simulink model "TST_Rail_BlkShtCtl"  (R2016b)
settings: Solver=FixedStepDiscrete  StartTime=0.0  StopTime=simTime  FixedStep=sampleTime  RelTol=1e-3
values from neighbouring files (symbols this model uses):
  testCase = 1    [initTST_Rail_BlkShtCtl_001.m]    (also in initTST_Rail_BlkShtCtl_002.m = 2; initTST_Rail_BlkShtCtl_003.m = 3)
libraries: simulink x7, UnitTest_Lib x3
settings Model: Creator=zhengjinyan  LastModifiedBy=zhengjinyan
settings DebuggingCC: SignalRangeChecking=error

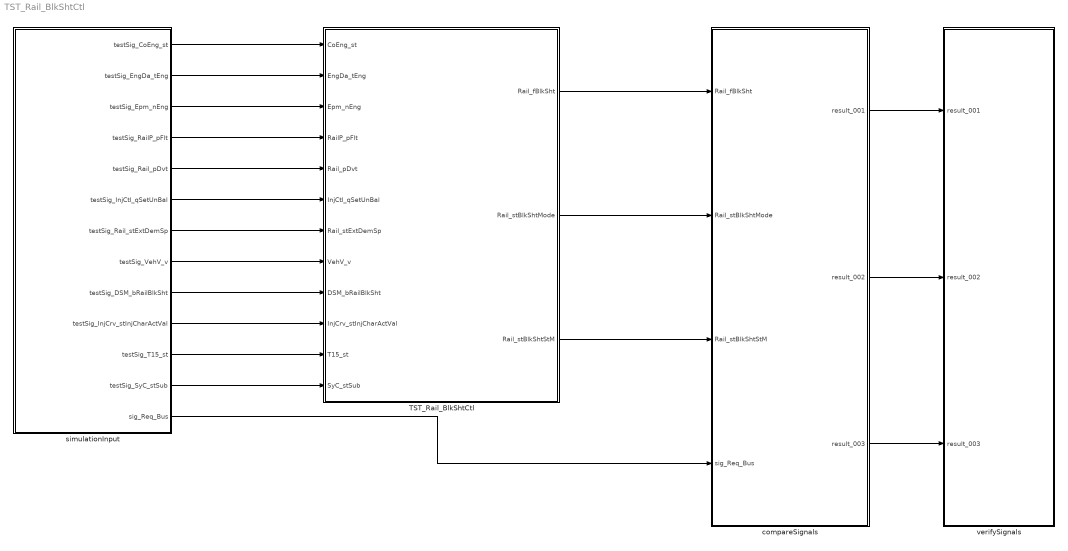
== system TST_Rail_BlkShtCtl ==
  TST_Rail_BlkShtCtl : Subsystem
  compareSignals : Subsystem
  simulationInput : Subsystem
  verifySignals : Subsystem
  wires:
  simulationInput/1(testSig_CoEng_st) -> TST_Rail_BlkShtCtl/1(CoEng_st)
  simulationInput/2(testSig_EngDa_tEng) -> TST_Rail_BlkShtCtl/2(EngDa_tEng)
  simulationInput/3(testSig_Epm_nEng) -> TST_Rail_BlkShtCtl/3(Epm_nEng)
  simulationInput/4(testSig_RailP_pFlt) -> TST_Rail_BlkShtCtl/4(RailP_pFlt)
  simulationInput/5(testSig_Rail_pDvt) -> TST_Rail_BlkShtCtl/5(Rail_pDvt)
  simulationInput/6(testSig_InjCtl_qSetUnBal) -> TST_Rail_BlkShtCtl/6(InjCtl_qSetUnBal)
  simulationInput/7(testSig_Rail_stExtDemSp) -> TST_Rail_BlkShtCtl/7(Rail_stExtDemSp)
  simulationInput/8(testSig_VehV_v) -> TST_Rail_BlkShtCtl/8(VehV_v)
  simulationInput/9(testSig_DSM_bRailBlkSht) -> TST_Rail_BlkShtCtl/9(DSM_bRailBlkSht)
  simulationInput/10(testSig_InjCrv_stInjCharActVal) -> TST_Rail_BlkShtCtl/10(InjCrv_stInjCharActVal)
  simulationInput/11(testSig_T15_st) -> TST_Rail_BlkShtCtl/11(T15_st)
  simulationInput/12(testSig_SyC_stSub) -> TST_Rail_BlkShtCtl/12(SyC_stSub)
  TST_Rail_BlkShtCtl/1(Rail_fBlkSht) -> compareSignals/1(Rail_fBlkSht)
  TST_Rail_BlkShtCtl/2(Rail_stBlkShtMode) -> compareSignals/2(Rail_stBlkShtMode)
  TST_Rail_BlkShtCtl/3(Rail_stBlkShtStM) -> compareSignals/3(Rail_stBlkShtStM)
  simulationInput/13(sig_Req_Bus) -> compareSignals/4(sig_Req_Bus)
  compareSignals/1(result_001) -> verifySignals/1(result_001)
  compareSignals/2(result_002) -> verifySignals/2(result_002)
  compareSignals/3(result_003) -> verifySignals/3(result_003)

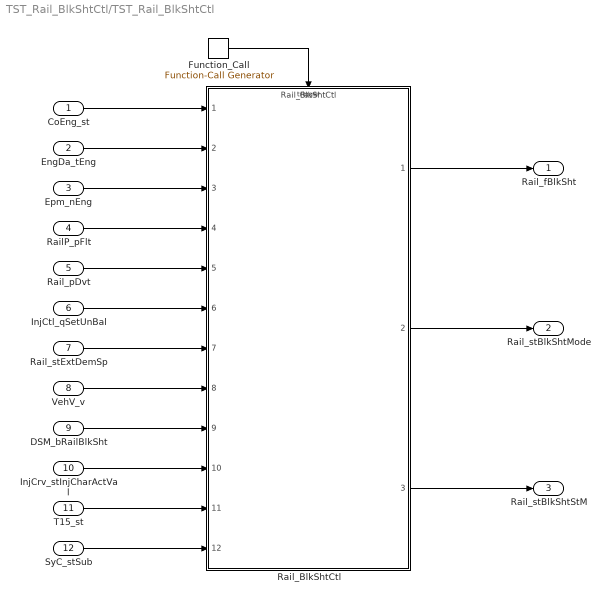
== system TST_Rail_BlkShtCtl/TST_Rail_BlkShtCtl ==
  CoEng_st : Inport
  EngDa_tEng : Inport  Port=2
  Epm_nEng : Inport  Port=3
  RailP_pFlt : Inport  Port=4
  Rail_pDvt : Inport  Port=5
  InjCtl_qSetUnBal : Inport  Port=6
  Rail_stExtDemSp : Inport  Port=7
  VehV_v : Inport  Port=8
  DSM_bRailBlkSht : Inport  Port=9
  InjCrv_stInjCharActVal : Inport  Port=10
  T15_st : Inport  Port=11
  SyC_stSub : Inport  Port=12
  Function_Call : simulink/Ports & Subsystems/Function-Call Generator  sample_time=sampleTime  numberOfIterations=1
  Rail_BlkShtCtl : ModelReference  ModelNameDialog=Rail_BlkShtCtl  SimulationMode=Normal  ModelReferenceVersion=1.164  TriggerPortName=function  TriggerPortTriggerType=function-call  TriggerPortStatesWhenEnabling=held
  Rail_fBlkSht : Outport
  Rail_stBlkShtMode : Outport  Port=2
  Rail_stBlkShtStM : Outport  Port=3
  wires:
  Function_Call/1 -> Rail_BlkShtCtl/Trigger
  CoEng_st/1 -> Rail_BlkShtCtl/1
  EngDa_tEng/1 -> Rail_BlkShtCtl/2
  Epm_nEng/1 -> Rail_BlkShtCtl/3
  RailP_pFlt/1 -> Rail_BlkShtCtl/4
  Rail_pDvt/1 -> Rail_BlkShtCtl/5
  InjCtl_qSetUnBal/1 -> Rail_BlkShtCtl/6
  Rail_stExtDemSp/1 -> Rail_BlkShtCtl/7
  VehV_v/1 -> Rail_BlkShtCtl/8
  DSM_bRailBlkSht/1 -> Rail_BlkShtCtl/9
  InjCrv_stInjCharActVal/1 -> Rail_BlkShtCtl/10
  T15_st/1 -> Rail_BlkShtCtl/11
  SyC_stSub/1 -> Rail_BlkShtCtl/12
  Rail_BlkShtCtl/1 -> Rail_fBlkSht/1
  Rail_BlkShtCtl/2 -> Rail_stBlkShtMode/1
  Rail_BlkShtCtl/3 -> Rail_stBlkShtStM/1

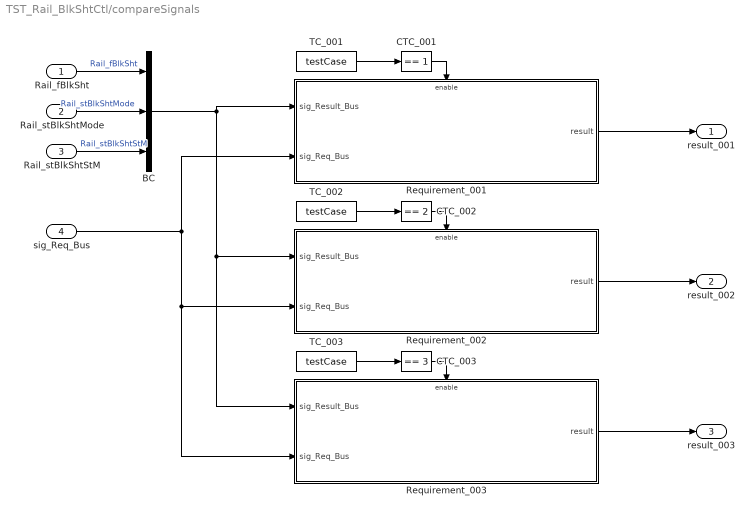
== system TST_Rail_BlkShtCtl/compareSignals ==
  Rail_fBlkSht : Inport
  Rail_stBlkShtMode : Inport  Port=2
  Rail_stBlkShtStM : Inport  Port=3
  sig_Req_Bus : Inport  Port=4
  BC : BusCreator  Inputs=3
  CTC_001 : simulink/Logic and Bit Operations/Compare To Constant  relop===  const=1  OutDataTypeStr=boolean
  CTC_002 : simulink/Logic and Bit Operations/Compare To Constant  relop===  const=2  OutDataTypeStr=boolean
  CTC_003 : simulink/Logic and Bit Operations/Compare To Constant  relop===  const=3  OutDataTypeStr=boolean
  Requirement_001 : Subsystem
  Requirement_002 : Subsystem
  Requirement_003 : Subsystem
  TC_001 : Constant  Value=testCase
  TC_002 : Constant  Value=testCase
  TC_003 : Constant  Value=testCase
  result_001 : Outport
  result_002 : Outport  Port=2
  result_003 : Outport  Port=3
  wires:
  Rail_fBlkSht/1 -> BC/1  "Rail_fBlkSht"
  Rail_stBlkShtMode/1 -> BC/2  "Rail_stBlkShtMode"
  Rail_stBlkShtStM/1 -> BC/3  "Rail_stBlkShtStM"
  TC_001/1 -> CTC_001/1
  CTC_001/1 -> Requirement_001/Enable
  sig_Req_Bus/1 -> Requirement_002/2(sig_Req_Bus), Requirement_003/2(sig_Req_Bus), Requirement_001/2(sig_Req_Bus)
  BC/1 -> Requirement_002/1(sig_Result_Bus), Requirement_003/1(sig_Result_Bus), Requirement_001/1(sig_Result_Bus)
  Requirement_001/1(result) -> result_001/1
  TC_002/1 -> CTC_002/1
  CTC_002/1 -> Requirement_002/Enable
  Requirement_002/1(result) -> result_002/1
  TC_003/1 -> CTC_003/1
  CTC_003/1 -> Requirement_003/Enable
  Requirement_003/1(result) -> result_003/1

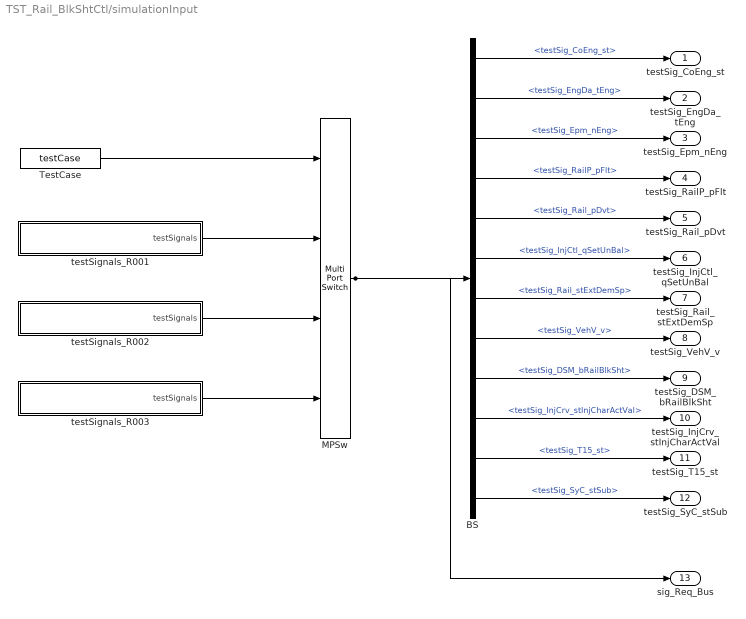
== system TST_Rail_BlkShtCtl/simulationInput ==
  BS : BusSelector  OutputSignals=testSig_CoEng_st,testSig_EngDa_tEng,testSig_Epm_nEng,testSig_RailP_pFlt,testSig_Rail_pDvt,testSig_InjCtl_qSetUnBal,testSig_Rail_stExtDemSp,testSig_VehV_v,testSig_DSM_bRailBlkSht,testSig_InjCrv_stInjCharActVal,testSig_T15_st,testSig_SyC_stSub
  MPSw : MultiPortSwitch  SaturateOnIntegerOverflow=on  InputSameDT=on
  TestCase : Constant  Value=testCase
  testSignals_R001 : Subsystem
  testSignals_R002 : Subsystem
  testSignals_R003 : Subsystem
  testSig_CoEng_st : Outport
  testSig_EngDa_tEng : Outport  Port=2
  testSig_Epm_nEng : Outport  Port=3
  testSig_RailP_pFlt : Outport  Port=4
  testSig_Rail_pDvt : Outport  Port=5
  testSig_InjCtl_qSetUnBal : Outport  Port=6
  testSig_Rail_stExtDemSp : Outport  Port=7
  testSig_VehV_v : Outport  Port=8
  testSig_DSM_bRailBlkSht : Outport  Port=9
  testSig_InjCrv_stInjCharActVal : Outport  Port=10
  testSig_T15_st : Outport  Port=11
  testSig_SyC_stSub : Outport  Port=12
  sig_Req_Bus : Outport  Port=13
  wires:
  BS/1 -> testSig_CoEng_st/1  "<testSig_CoEng_st>"
  BS/2 -> testSig_EngDa_tEng/1  "<testSig_EngDa_tEng>"
  BS/3 -> testSig_Epm_nEng/1  "<testSig_Epm_nEng>"
  BS/4 -> testSig_RailP_pFlt/1  "<testSig_RailP_pFlt>"
  BS/5 -> testSig_Rail_pDvt/1  "<testSig_Rail_pDvt>"
  BS/6 -> testSig_InjCtl_qSetUnBal/1  "<testSig_InjCtl_qSetUnBal>"
  BS/7 -> testSig_Rail_stExtDemSp/1  "<testSig_Rail_stExtDemSp>"
  BS/8 -> testSig_VehV_v/1  "<testSig_VehV_v>"
  BS/9 -> testSig_DSM_bRailBlkSht/1  "<testSig_DSM_bRailBlkSht>"
  BS/10 -> testSig_InjCrv_stInjCharActVal/1  "<testSig_InjCrv_stInjCharActVal>"
  BS/11 -> testSig_T15_st/1  "<testSig_T15_st>"
  BS/12 -> testSig_SyC_stSub/1  "<testSig_SyC_stSub>"
  MPSw/1 -> BS/1, sig_Req_Bus/1
  TestCase/1 -> MPSw/1
  testSignals_R001/1(testSignals) -> MPSw/2
  testSignals_R002/1(testSignals) -> MPSw/3
  testSignals_R003/1(testSignals) -> MPSw/4

== system TST_Rail_BlkShtCtl/verifySignals ==
  result_001 : Inport
  result_002 : Inport  Port=2
  result_003 : Inport  Port=3
  Assertion_001 : Assertion  Enabled=off
  Assertion_002 : Assertion  Enabled=off
  Assertion_003 : Assertion  Enabled=off
  wires:
  result_001/1 -> Assertion_001/1
  result_002/1 -> Assertion_002/1
  result_003/1 -> Assertion_003/1

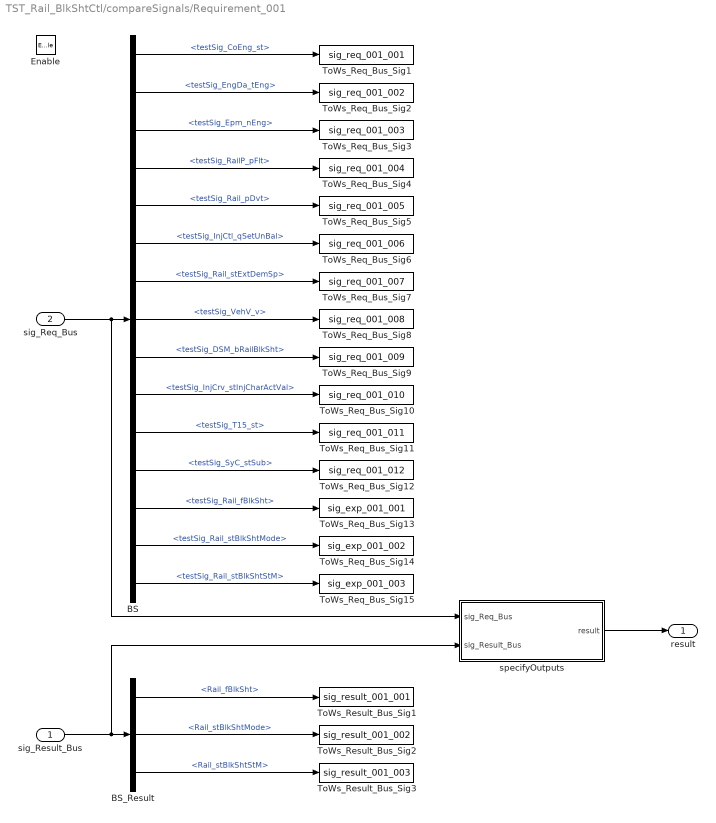
== system TST_Rail_BlkShtCtl/compareSignals/Requirement_001 ==
  sig_Result_Bus : Inport
  sig_Req_Bus : Inport  Port=2
  Enable : EnablePort
  BS : BusSelector  OutputSignals=testSig_CoEng_st,testSig_EngDa_tEng,testSig_Epm_nEng,testSig_RailP_pFlt,testSig_Rail_pDvt,testSig_InjCtl_qSetUnBal,testSig_Rail_stExtDemSp,testSig_VehV_v,testSig_DSM_bRailBlkSht,testSig_InjCrv_stInjCharActVal,testSig_T15_st,testSig_SyC_stSub,testSig_Rail_fBlkSht,testSig_Rail_stBlkShtMode,testSig_Rail_stBlkShtStM
  BS_Result : BusSelector  OutputSignals=Rail_fBlkSht,Rail_stBlkShtMode,Rail_stBlkShtStM
  ToWs_Req_Bus_Sig1 : ToWorkspace  VariableName=sig_req_001_001  SaveFormat=Structure With Time
  ToWs_Req_Bus_Sig10 : ToWorkspace  VariableName=sig_req_001_010  SaveFormat=Structure With Time
  ToWs_Req_Bus_Sig11 : ToWorkspace  VariableName=sig_req_001_011  SaveFormat=Structure With Time
  ToWs_Req_Bus_Sig12 : ToWorkspace  VariableName=sig_req_001_012  SaveFormat=Structure With Time
  ToWs_Req_Bus_Sig13 : ToWorkspace  VariableName=sig_exp_001_001  SaveFormat=Structure With Time
  ToWs_Req_Bus_Sig14 : ToWorkspace  VariableName=sig_exp_001_002  SaveFormat=Structure With Time
  ToWs_Req_Bus_Sig15 : ToWorkspace  VariableName=sig_exp_001_003  SaveFormat=Structure With Time
  ToWs_Req_Bus_Sig2 : ToWorkspace  VariableName=sig_req_001_002  SaveFormat=Structure With Time
  ToWs_Req_Bus_Sig3 : ToWorkspace  VariableName=sig_req_001_003  SaveFormat=Structure With Time
  ToWs_Req_Bus_Sig4 : ToWorkspace  VariableName=sig_req_001_004  SaveFormat=Structure With Time
  ToWs_Req_Bus_Sig5 : ToWorkspace  VariableName=sig_req_001_005  SaveFormat=Structure With Time
  ToWs_Req_Bus_Sig6 : ToWorkspace  VariableName=sig_req_001_006  SaveFormat=Structure With Time
  ToWs_Req_Bus_Sig7 : ToWorkspace  VariableName=sig_req_001_007  SaveFormat=Structure With Time
  ToWs_Req_Bus_Sig8 : ToWorkspace  VariableName=sig_req_001_008  SaveFormat=Structure With Time
  ToWs_Req_Bus_Sig9 : ToWorkspace  VariableName=sig_req_001_009  SaveFormat=Structure With Time
  ToWs_Result_Bus_Sig1 : ToWorkspace  VariableName=sig_result_001_001  SaveFormat=Structure With Time
  ToWs_Result_Bus_Sig2 : ToWorkspace  VariableName=sig_result_001_002  SaveFormat=Structure With Time
  ToWs_Result_Bus_Sig3 : ToWorkspace  VariableName=sig_result_001_003  SaveFormat=Structure With Time
  specifyOutputs : Subsystem
  result : Outport
  wires:
  sig_Req_Bus/1 -> BS/1, specifyOutputs/1(sig_Req_Bus)
  BS/1 -> ToWs_Req_Bus_Sig1/1  "<testSig_CoEng_st>"
  BS/2 -> ToWs_Req_Bus_Sig2/1  "<testSig_EngDa_tEng>"
  BS/3 -> ToWs_Req_Bus_Sig3/1  "<testSig_Epm_nEng>"
  BS/4 -> ToWs_Req_Bus_Sig4/1  "<testSig_RailP_pFlt>"
  BS/5 -> ToWs_Req_Bus_Sig5/1  "<testSig_Rail_pDvt>"
  BS/6 -> ToWs_Req_Bus_Sig6/1  "<testSig_InjCtl_qSetUnBal>"
  BS/7 -> ToWs_Req_Bus_Sig7/1  "<testSig_Rail_stExtDemSp>"
  BS/8 -> ToWs_Req_Bus_Sig8/1  "<testSig_VehV_v>"
  BS/9 -> ToWs_Req_Bus_Sig9/1  "<testSig_DSM_bRailBlkSht>"
  BS/10 -> ToWs_Req_Bus_Sig10/1  "<testSig_InjCrv_stInjCharActVal>"
  BS/11 -> ToWs_Req_Bus_Sig11/1  "<testSig_T15_st>"
  BS/12 -> ToWs_Req_Bus_Sig12/1  "<testSig_SyC_stSub>"
  BS/13 -> ToWs_Req_Bus_Sig13/1  "<testSig_Rail_fBlkSht>"
  BS/14 -> ToWs_Req_Bus_Sig14/1  "<testSig_Rail_stBlkShtMode>"
  BS/15 -> ToWs_Req_Bus_Sig15/1  "<testSig_Rail_stBlkShtStM>"
  sig_Result_Bus/1 -> BS_Result/1, specifyOutputs/2(sig_Result_Bus)
  BS_Result/1 -> ToWs_Result_Bus_Sig1/1  "<Rail_fBlkSht>"
  BS_Result/2 -> ToWs_Result_Bus_Sig2/1  "<Rail_stBlkShtMode>"
  BS_Result/3 -> ToWs_Result_Bus_Sig3/1  "<Rail_stBlkShtStM>"
  specifyOutputs/1(result) -> result/1

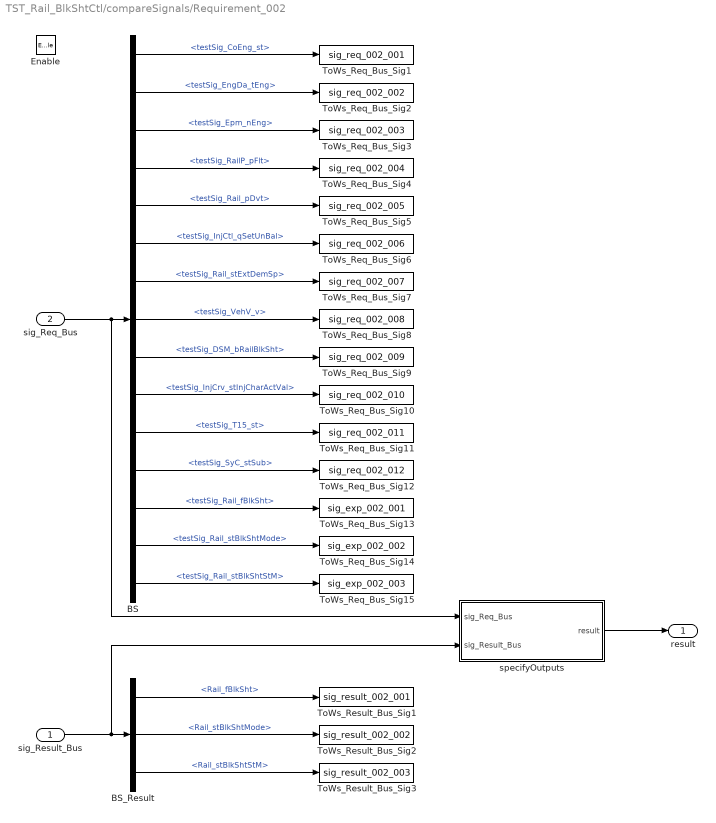
== system TST_Rail_BlkShtCtl/compareSignals/Requirement_002 ==
  sig_Result_Bus : Inport
  sig_Req_Bus : Inport  Port=2
  Enable : EnablePort
  BS : BusSelector  OutputSignals=testSig_CoEng_st,testSig_EngDa_tEng,testSig_Epm_nEng,testSig_RailP_pFlt,testSig_Rail_pDvt,testSig_InjCtl_qSetUnBal,testSig_Rail_stExtDemSp,testSig_VehV_v,testSig_DSM_bRailBlkSht,testSig_InjCrv_stInjCharActVal,testSig_T15_st,testSig_SyC_stSub,testSig_Rail_fBlkSht,testSig_Rail_stBlkShtMode,testSig_Rail_stBlkShtStM
  BS_Result : BusSelector  OutputSignals=Rail_fBlkSht,Rail_stBlkShtMode,Rail_stBlkShtStM
  ToWs_Req_Bus_Sig1 : ToWorkspace  VariableName=sig_req_002_001  SaveFormat=Structure With Time
  ToWs_Req_Bus_Sig10 : ToWorkspace  VariableName=sig_req_002_010  SaveFormat=Structure With Time
  ToWs_Req_Bus_Sig11 : ToWorkspace  VariableName=sig_req_002_011  SaveFormat=Structure With Time
  ToWs_Req_Bus_Sig12 : ToWorkspace  VariableName=sig_req_002_012  SaveFormat=Structure With Time
  ToWs_Req_Bus_Sig13 : ToWorkspace  VariableName=sig_exp_002_001  SaveFormat=Structure With Time
  ToWs_Req_Bus_Sig14 : ToWorkspace  VariableName=sig_exp_002_002  SaveFormat=Structure With Time
  ToWs_Req_Bus_Sig15 : ToWorkspace  VariableName=sig_exp_002_003  SaveFormat=Structure With Time
  ToWs_Req_Bus_Sig2 : ToWorkspace  VariableName=sig_req_002_002  SaveFormat=Structure With Time
  ToWs_Req_Bus_Sig3 : ToWorkspace  VariableName=sig_req_002_003  SaveFormat=Structure With Time
  ToWs_Req_Bus_Sig4 : ToWorkspace  VariableName=sig_req_002_004  SaveFormat=Structure With Time
  ToWs_Req_Bus_Sig5 : ToWorkspace  VariableName=sig_req_002_005  SaveFormat=Structure With Time
  ToWs_Req_Bus_Sig6 : ToWorkspace  VariableName=sig_req_002_006  SaveFormat=Structure With Time
  ToWs_Req_Bus_Sig7 : ToWorkspace  VariableName=sig_req_002_007  SaveFormat=Structure With Time
  ToWs_Req_Bus_Sig8 : ToWorkspace  VariableName=sig_req_002_008  SaveFormat=Structure With Time
  ToWs_Req_Bus_Sig9 : ToWorkspace  VariableName=sig_req_002_009  SaveFormat=Structure With Time
  ToWs_Result_Bus_Sig1 : ToWorkspace  VariableName=sig_result_002_001  SaveFormat=Structure With Time
  ToWs_Result_Bus_Sig2 : ToWorkspace  VariableName=sig_result_002_002  SaveFormat=Structure With Time
  ToWs_Result_Bus_Sig3 : ToWorkspace  VariableName=sig_result_002_003  SaveFormat=Structure With Time
  specifyOutputs : Subsystem
  result : Outport
  wires:
  sig_Req_Bus/1 -> BS/1, specifyOutputs/1(sig_Req_Bus)
  BS/1 -> ToWs_Req_Bus_Sig1/1  "<testSig_CoEng_st>"
  BS/2 -> ToWs_Req_Bus_Sig2/1  "<testSig_EngDa_tEng>"
  BS/3 -> ToWs_Req_Bus_Sig3/1  "<testSig_Epm_nEng>"
  BS/4 -> ToWs_Req_Bus_Sig4/1  "<testSig_RailP_pFlt>"
  BS/5 -> ToWs_Req_Bus_Sig5/1  "<testSig_Rail_pDvt>"
  BS/6 -> ToWs_Req_Bus_Sig6/1  "<testSig_InjCtl_qSetUnBal>"
  BS/7 -> ToWs_Req_Bus_Sig7/1  "<testSig_Rail_stExtDemSp>"
  BS/8 -> ToWs_Req_Bus_Sig8/1  "<testSig_VehV_v>"
  BS/9 -> ToWs_Req_Bus_Sig9/1  "<testSig_DSM_bRailBlkSht>"
  BS/10 -> ToWs_Req_Bus_Sig10/1  "<testSig_InjCrv_stInjCharActVal>"
  BS/11 -> ToWs_Req_Bus_Sig11/1  "<testSig_T15_st>"
  BS/12 -> ToWs_Req_Bus_Sig12/1  "<testSig_SyC_stSub>"
  BS/13 -> ToWs_Req_Bus_Sig13/1  "<testSig_Rail_fBlkSht>"
  BS/14 -> ToWs_Req_Bus_Sig14/1  "<testSig_Rail_stBlkShtMode>"
  BS/15 -> ToWs_Req_Bus_Sig15/1  "<testSig_Rail_stBlkShtStM>"
  sig_Result_Bus/1 -> BS_Result/1, specifyOutputs/2(sig_Result_Bus)
  BS_Result/1 -> ToWs_Result_Bus_Sig1/1  "<Rail_fBlkSht>"
  BS_Result/2 -> ToWs_Result_Bus_Sig2/1  "<Rail_stBlkShtMode>"
  BS_Result/3 -> ToWs_Result_Bus_Sig3/1  "<Rail_stBlkShtStM>"
  specifyOutputs/1(result) -> result/1

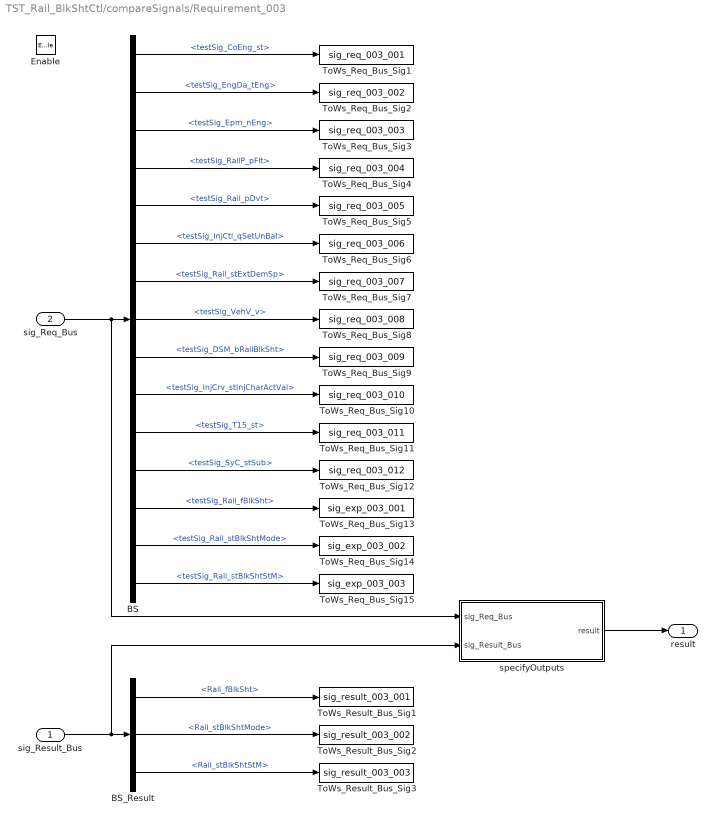
== system TST_Rail_BlkShtCtl/compareSignals/Requirement_003 ==
  sig_Result_Bus : Inport
  sig_Req_Bus : Inport  Port=2
  Enable : EnablePort
  BS : BusSelector  OutputSignals=testSig_CoEng_st,testSig_EngDa_tEng,testSig_Epm_nEng,testSig_RailP_pFlt,testSig_Rail_pDvt,testSig_InjCtl_qSetUnBal,testSig_Rail_stExtDemSp,testSig_VehV_v,testSig_DSM_bRailBlkSht,testSig_InjCrv_stInjCharActVal,testSig_T15_st,testSig_SyC_stSub,testSig_Rail_fBlkSht,testSig_Rail_stBlkShtMode,testSig_Rail_stBlkShtStM
  BS_Result : BusSelector  OutputSignals=Rail_fBlkSht,Rail_stBlkShtMode,Rail_stBlkShtStM
  ToWs_Req_Bus_Sig1 : ToWorkspace  VariableName=sig_req_003_001  SaveFormat=Structure With Time
  ToWs_Req_Bus_Sig10 : ToWorkspace  VariableName=sig_req_003_010  SaveFormat=Structure With Time
  ToWs_Req_Bus_Sig11 : ToWorkspace  VariableName=sig_req_003_011  SaveFormat=Structure With Time
  ToWs_Req_Bus_Sig12 : ToWorkspace  VariableName=sig_req_003_012  SaveFormat=Structure With Time
  ToWs_Req_Bus_Sig13 : ToWorkspace  VariableName=sig_exp_003_001  SaveFormat=Structure With Time
  ToWs_Req_Bus_Sig14 : ToWorkspace  VariableName=sig_exp_003_002  SaveFormat=Structure With Time
  ToWs_Req_Bus_Sig15 : ToWorkspace  VariableName=sig_exp_003_003  SaveFormat=Structure With Time
  ToWs_Req_Bus_Sig2 : ToWorkspace  VariableName=sig_req_003_002  SaveFormat=Structure With Time
  ToWs_Req_Bus_Sig3 : ToWorkspace  VariableName=sig_req_003_003  SaveFormat=Structure With Time
  ToWs_Req_Bus_Sig4 : ToWorkspace  VariableName=sig_req_003_004  SaveFormat=Structure With Time
  ToWs_Req_Bus_Sig5 : ToWorkspace  VariableName=sig_req_003_005  SaveFormat=Structure With Time
  ToWs_Req_Bus_Sig6 : ToWorkspace  VariableName=sig_req_003_006  SaveFormat=Structure With Time
  ToWs_Req_Bus_Sig7 : ToWorkspace  VariableName=sig_req_003_007  SaveFormat=Structure With Time
  ToWs_Req_Bus_Sig8 : ToWorkspace  VariableName=sig_req_003_008  SaveFormat=Structure With Time
  ToWs_Req_Bus_Sig9 : ToWorkspace  VariableName=sig_req_003_009  SaveFormat=Structure With Time
  ToWs_Result_Bus_Sig1 : ToWorkspace  VariableName=sig_result_003_001  SaveFormat=Structure With Time
  ToWs_Result_Bus_Sig2 : ToWorkspace  VariableName=sig_result_003_002  SaveFormat=Structure With Time
  ToWs_Result_Bus_Sig3 : ToWorkspace  VariableName=sig_result_003_003  SaveFormat=Structure With Time
  specifyOutputs : Subsystem
  result : Outport
  wires:
  sig_Req_Bus/1 -> BS/1, specifyOutputs/1(sig_Req_Bus)
  BS/1 -> ToWs_Req_Bus_Sig1/1  "<testSig_CoEng_st>"
  BS/2 -> ToWs_Req_Bus_Sig2/1  "<testSig_EngDa_tEng>"
  BS/3 -> ToWs_Req_Bus_Sig3/1  "<testSig_Epm_nEng>"
  BS/4 -> ToWs_Req_Bus_Sig4/1  "<testSig_RailP_pFlt>"
  BS/5 -> ToWs_Req_Bus_Sig5/1  "<testSig_Rail_pDvt>"
  BS/6 -> ToWs_Req_Bus_Sig6/1  "<testSig_InjCtl_qSetUnBal>"
  BS/7 -> ToWs_Req_Bus_Sig7/1  "<testSig_Rail_stExtDemSp>"
  BS/8 -> ToWs_Req_Bus_Sig8/1  "<testSig_VehV_v>"
  BS/9 -> ToWs_Req_Bus_Sig9/1  "<testSig_DSM_bRailBlkSht>"
  BS/10 -> ToWs_Req_Bus_Sig10/1  "<testSig_InjCrv_stInjCharActVal>"
  BS/11 -> ToWs_Req_Bus_Sig11/1  "<testSig_T15_st>"
  BS/12 -> ToWs_Req_Bus_Sig12/1  "<testSig_SyC_stSub>"
  BS/13 -> ToWs_Req_Bus_Sig13/1  "<testSig_Rail_fBlkSht>"
  BS/14 -> ToWs_Req_Bus_Sig14/1  "<testSig_Rail_stBlkShtMode>"
  BS/15 -> ToWs_Req_Bus_Sig15/1  "<testSig_Rail_stBlkShtStM>"
  sig_Result_Bus/1 -> BS_Result/1, specifyOutputs/2(sig_Result_Bus)
  BS_Result/1 -> ToWs_Result_Bus_Sig1/1  "<Rail_fBlkSht>"
  BS_Result/2 -> ToWs_Result_Bus_Sig2/1  "<Rail_stBlkShtMode>"
  BS_Result/3 -> ToWs_Result_Bus_Sig3/1  "<Rail_stBlkShtStM>"
  specifyOutputs/1(result) -> result/1

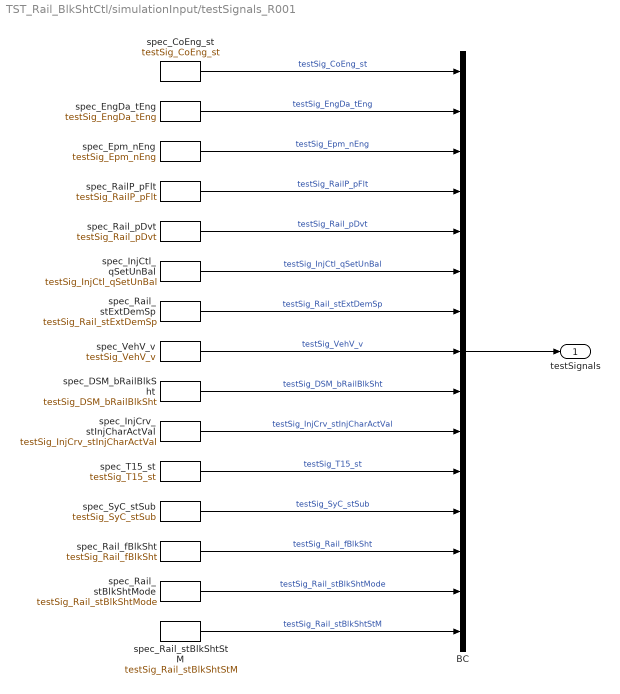
== system TST_Rail_BlkShtCtl/simulationInput/testSignals_R001 ==
  BC : BusCreator  Inputs=15
  spec_CoEng_st : FromWorkspace  VariableName=testSig_CoEng_st  Interpolate=off  OutputAfterFinalValue=Holding final value
  spec_DSM_bRailBlkSht : FromWorkspace  VariableName=testSig_DSM_bRailBlkSht  Interpolate=off  OutputAfterFinalValue=Holding final value
  spec_EngDa_tEng : FromWorkspace  VariableName=testSig_EngDa_tEng  Interpolate=off  OutputAfterFinalValue=Holding final value
  spec_Epm_nEng : FromWorkspace  VariableName=testSig_Epm_nEng  Interpolate=off  OutputAfterFinalValue=Holding final value
  spec_InjCrv_stInjCharActVal : FromWorkspace  VariableName=testSig_InjCrv_stInjCharActVal  Interpolate=off  OutputAfterFinalValue=Holding final value
  spec_InjCtl_qSetUnBal : FromWorkspace  VariableName=testSig_InjCtl_qSetUnBal  Interpolate=off  OutputAfterFinalValue=Holding final value
  spec_RailP_pFlt : FromWorkspace  VariableName=testSig_RailP_pFlt  Interpolate=off  OutputAfterFinalValue=Holding final value
  spec_Rail_fBlkSht : FromWorkspace  VariableName=testSig_Rail_fBlkSht  Interpolate=off  OutputAfterFinalValue=Holding final value
  spec_Rail_pDvt : FromWorkspace  VariableName=testSig_Rail_pDvt  Interpolate=off  OutputAfterFinalValue=Holding final value
  spec_Rail_stBlkShtMode : FromWorkspace  VariableName=testSig_Rail_stBlkShtMode  Interpolate=off  OutputAfterFinalValue=Holding final value
  spec_Rail_stBlkShtStM : FromWorkspace  VariableName=testSig_Rail_stBlkShtStM  Interpolate=off  OutputAfterFinalValue=Holding final value
  spec_Rail_stExtDemSp : FromWorkspace  VariableName=testSig_Rail_stExtDemSp  Interpolate=off  OutputAfterFinalValue=Holding final value
  spec_SyC_stSub : FromWorkspace  VariableName=testSig_SyC_stSub  Interpolate=off  OutputAfterFinalValue=Holding final value
  spec_T15_st : FromWorkspace  VariableName=testSig_T15_st  Interpolate=off  OutputAfterFinalValue=Holding final value
  spec_VehV_v : FromWorkspace  VariableName=testSig_VehV_v  Interpolate=off  OutputAfterFinalValue=Holding final value
  testSignals : Outport
  wires:
  BC/1 -> testSignals/1
  spec_CoEng_st/1 -> BC/1  "testSig_CoEng_st"
  spec_EngDa_tEng/1 -> BC/2  "testSig_EngDa_tEng"
  spec_Epm_nEng/1 -> BC/3  "testSig_Epm_nEng"
  spec_RailP_pFlt/1 -> BC/4  "testSig_RailP_pFlt"
  spec_Rail_pDvt/1 -> BC/5  "testSig_Rail_pDvt"
  spec_InjCtl_qSetUnBal/1 -> BC/6  "testSig_InjCtl_qSetUnBal"
  spec_Rail_stExtDemSp/1 -> BC/7  "testSig_Rail_stExtDemSp"
  spec_VehV_v/1 -> BC/8  "testSig_VehV_v"
  spec_DSM_bRailBlkSht/1 -> BC/9  "testSig_DSM_bRailBlkSht"
  spec_InjCrv_stInjCharActVal/1 -> BC/10  "testSig_InjCrv_stInjCharActVal"
  spec_T15_st/1 -> BC/11  "testSig_T15_st"
  spec_SyC_stSub/1 -> BC/12  "testSig_SyC_stSub"
  spec_Rail_fBlkSht/1 -> BC/13  "testSig_Rail_fBlkSht"
  spec_Rail_stBlkShtMode/1 -> BC/14  "testSig_Rail_stBlkShtMode"
  spec_Rail_stBlkShtStM/1 -> BC/15  "testSig_Rail_stBlkShtStM"

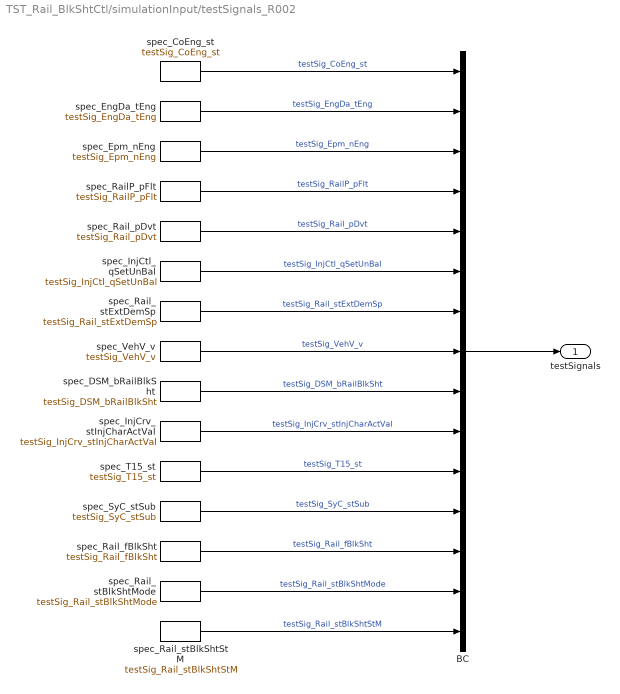
== system TST_Rail_BlkShtCtl/simulationInput/testSignals_R002 ==
  BC : BusCreator  Inputs=15
  spec_CoEng_st : FromWorkspace  VariableName=testSig_CoEng_st  Interpolate=off  OutputAfterFinalValue=Holding final value
  spec_DSM_bRailBlkSht : FromWorkspace  VariableName=testSig_DSM_bRailBlkSht  Interpolate=off  OutputAfterFinalValue=Holding final value
  spec_EngDa_tEng : FromWorkspace  VariableName=testSig_EngDa_tEng  Interpolate=off  OutputAfterFinalValue=Holding final value
  spec_Epm_nEng : FromWorkspace  VariableName=testSig_Epm_nEng  Interpolate=off  OutputAfterFinalValue=Holding final value
  spec_InjCrv_stInjCharActVal : FromWorkspace  VariableName=testSig_InjCrv_stInjCharActVal  Interpolate=off  OutputAfterFinalValue=Holding final value
  spec_InjCtl_qSetUnBal : FromWorkspace  VariableName=testSig_InjCtl_qSetUnBal  Interpolate=off  OutputAfterFinalValue=Holding final value
  spec_RailP_pFlt : FromWorkspace  VariableName=testSig_RailP_pFlt  Interpolate=off  OutputAfterFinalValue=Holding final value
  spec_Rail_fBlkSht : FromWorkspace  VariableName=testSig_Rail_fBlkSht  Interpolate=off  OutputAfterFinalValue=Holding final value
  spec_Rail_pDvt : FromWorkspace  VariableName=testSig_Rail_pDvt  Interpolate=off  OutputAfterFinalValue=Holding final value
  spec_Rail_stBlkShtMode : FromWorkspace  VariableName=testSig_Rail_stBlkShtMode  Interpolate=off  OutputAfterFinalValue=Holding final value
  spec_Rail_stBlkShtStM : FromWorkspace  VariableName=testSig_Rail_stBlkShtStM  Interpolate=off  OutputAfterFinalValue=Holding final value
  spec_Rail_stExtDemSp : FromWorkspace  VariableName=testSig_Rail_stExtDemSp  Interpolate=off  OutputAfterFinalValue=Holding final value
  spec_SyC_stSub : FromWorkspace  VariableName=testSig_SyC_stSub  Interpolate=off  OutputAfterFinalValue=Holding final value
  spec_T15_st : FromWorkspace  VariableName=testSig_T15_st  Interpolate=off  OutputAfterFinalValue=Holding final value
  spec_VehV_v : FromWorkspace  VariableName=testSig_VehV_v  Interpolate=off  OutputAfterFinalValue=Holding final value
  testSignals : Outport
  wires:
  BC/1 -> testSignals/1
  spec_CoEng_st/1 -> BC/1  "testSig_CoEng_st"
  spec_EngDa_tEng/1 -> BC/2  "testSig_EngDa_tEng"
  spec_Epm_nEng/1 -> BC/3  "testSig_Epm_nEng"
  spec_RailP_pFlt/1 -> BC/4  "testSig_RailP_pFlt"
  spec_Rail_pDvt/1 -> BC/5  "testSig_Rail_pDvt"
  spec_InjCtl_qSetUnBal/1 -> BC/6  "testSig_InjCtl_qSetUnBal"
  spec_Rail_stExtDemSp/1 -> BC/7  "testSig_Rail_stExtDemSp"
  spec_VehV_v/1 -> BC/8  "testSig_VehV_v"
  spec_DSM_bRailBlkSht/1 -> BC/9  "testSig_DSM_bRailBlkSht"
  spec_InjCrv_stInjCharActVal/1 -> BC/10  "testSig_InjCrv_stInjCharActVal"
  spec_T15_st/1 -> BC/11  "testSig_T15_st"
  spec_SyC_stSub/1 -> BC/12  "testSig_SyC_stSub"
  spec_Rail_fBlkSht/1 -> BC/13  "testSig_Rail_fBlkSht"
  spec_Rail_stBlkShtMode/1 -> BC/14  "testSig_Rail_stBlkShtMode"
  spec_Rail_stBlkShtStM/1 -> BC/15  "testSig_Rail_stBlkShtStM"

== system TST_Rail_BlkShtCtl/simulationInput/testSignals_R003 ==
  BC : BusCreator  Inputs=15
  spec_CoEng_st : FromWorkspace  VariableName=testSig_CoEng_st  Interpolate=off  OutputAfterFinalValue=Holding final value
  spec_DSM_bRailBlkSht : FromWorkspace  VariableName=testSig_DSM_bRailBlkSht  Interpolate=off  OutputAfterFinalValue=Holding final value
  spec_EngDa_tEng : FromWorkspace  VariableName=testSig_EngDa_tEng  Interpolate=off  OutputAfterFinalValue=Holding final value
  spec_Epm_nEng : FromWorkspace  VariableName=testSig_Epm_nEng  Interpolate=off  OutputAfterFinalValue=Holding final value
  spec_InjCrv_stInjCharActVal : FromWorkspace  VariableName=testSig_InjCrv_stInjCharActVal  Interpolate=off  OutputAfterFinalValue=Holding final value
  spec_InjCtl_qSetUnBal : FromWorkspace  VariableName=testSig_InjCtl_qSetUnBal  Interpolate=off  OutputAfterFinalValue=Holding final value
  spec_RailP_pFlt : FromWorkspace  VariableName=testSig_RailP_pFlt  Interpolate=off  OutputAfterFinalValue=Holding final value
  spec_Rail_fBlkSht : FromWorkspace  VariableName=testSig_Rail_fBlkSht  Interpolate=off  OutputAfterFinalValue=Holding final value
  spec_Rail_pDvt : FromWorkspace  VariableName=testSig_Rail_pDvt  Interpolate=off  OutputAfterFinalValue=Holding final value
  spec_Rail_stBlkShtMode : FromWorkspace  VariableName=testSig_Rail_stBlkShtMode  Interpolate=off  OutputAfterFinalValue=Holding final value
  spec_Rail_stBlkShtStM : FromWorkspace  VariableName=testSig_Rail_stBlkShtStM  Interpolate=off  OutputAfterFinalValue=Holding final value
  spec_Rail_stExtDemSp : FromWorkspace  VariableName=testSig_Rail_stExtDemSp  Interpolate=off  OutputAfterFinalValue=Holding final value
  spec_SyC_stSub : FromWorkspace  VariableName=testSig_SyC_stSub  Interpolate=off  OutputAfterFinalValue=Holding final value
  spec_T15_st : FromWorkspace  VariableName=testSig_T15_st  Interpolate=off  OutputAfterFinalValue=Holding final value
  spec_VehV_v : FromWorkspace  VariableName=testSig_VehV_v  Interpolate=off  OutputAfterFinalValue=Holding final value
  testSignals : Outport
  wires:
  BC/1 -> testSignals/1
  spec_CoEng_st/1 -> BC/1  "testSig_CoEng_st"
  spec_EngDa_tEng/1 -> BC/2  "testSig_EngDa_tEng"
  spec_Epm_nEng/1 -> BC/3  "testSig_Epm_nEng"
  spec_RailP_pFlt/1 -> BC/4  "testSig_RailP_pFlt"
  spec_Rail_pDvt/1 -> BC/5  "testSig_Rail_pDvt"
  spec_InjCtl_qSetUnBal/1 -> BC/6  "testSig_InjCtl_qSetUnBal"
  spec_Rail_stExtDemSp/1 -> BC/7  "testSig_Rail_stExtDemSp"
  spec_VehV_v/1 -> BC/8  "testSig_VehV_v"
  spec_DSM_bRailBlkSht/1 -> BC/9  "testSig_DSM_bRailBlkSht"
  spec_InjCrv_stInjCharActVal/1 -> BC/10  "testSig_InjCrv_stInjCharActVal"
  spec_T15_st/1 -> BC/11  "testSig_T15_st"
  spec_SyC_stSub/1 -> BC/12  "testSig_SyC_stSub"
  spec_Rail_fBlkSht/1 -> BC/13  "testSig_Rail_fBlkSht"
  spec_Rail_stBlkShtMode/1 -> BC/14  "testSig_Rail_stBlkShtMode"
  spec_Rail_stBlkShtStM/1 -> BC/15  "testSig_Rail_stBlkShtStM"

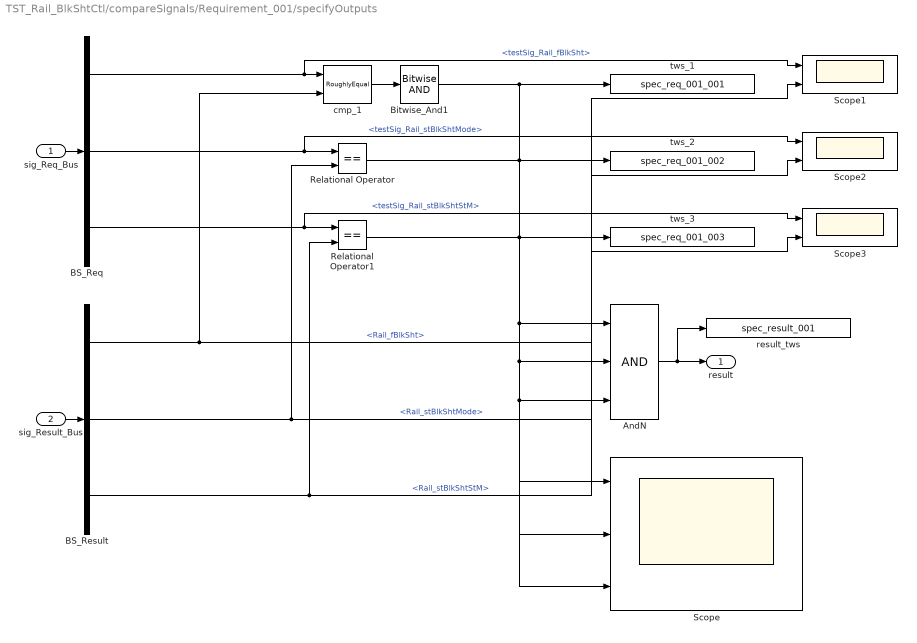
== system TST_Rail_BlkShtCtl/compareSignals/Requirement_001/specifyOutputs ==
  sig_Req_Bus : Inport
  sig_Result_Bus : Inport  Port=2
  AndN : Logic  Inputs=3
  BS_Req : BusSelector  OutputSignals=testSig_Rail_fBlkSht,testSig_Rail_stBlkShtMode,testSig_Rail_stBlkShtStM
  BS_Result : BusSelector  OutputSignals=Rail_fBlkSht,Rail_stBlkShtMode,Rail_stBlkShtStM
  Bitwise_And1 : simulink/Logic and Bit Operations/Bitwise Operator  logicop=AND  UseBitMask=off  BitMask=bin2dec('11011001')  BitMaskRealWorld=Stored Integer
  Relational Operator : RelationalOperator  Operator===  OutDataTypeStr=boolean  RndMeth=Simplest
  Relational Operator1 : RelationalOperator  Operator===  OutDataTypeStr=boolean  RndMeth=Simplest
  Scope : Scope  NumInputPorts=3
  Scope1 : Scope  NumInputPorts=2
  Scope2 : Scope  NumInputPorts=2
  Scope3 : Scope  NumInputPorts=2
  cmp_1 : UnitTest_Lib/RoughlyEqual  slope=0.1
  result_tws : ToWorkspace  VariableName=spec_result_001
  tws_1 : ToWorkspace  VariableName=spec_req_001_001
  tws_2 : ToWorkspace  VariableName=spec_req_001_002
  tws_3 : ToWorkspace  VariableName=spec_req_001_003
  result : Outport
  wires:
  sig_Req_Bus/1 -> BS_Req/1
  sig_Result_Bus/1 -> BS_Result/1
  AndN/1 -> result/1, result_tws/1
  BS_Req/1 -> cmp_1/1, Scope1/1  "<testSig_Rail_fBlkSht>"
  BS_Result/1 -> cmp_1/2, Scope1/2  "<Rail_fBlkSht>"
  cmp_1/1 -> Bitwise_And1/1
  Bitwise_And1/1 -> AndN/1, Scope/1, tws_1/1
  BS_Req/2 -> Relational Operator/1, Scope2/1  "<testSig_Rail_stBlkShtMode>"
  BS_Result/2 -> Scope2/2, Relational Operator/2  "<Rail_stBlkShtMode>"
  Relational Operator/1 -> AndN/2, Scope/2, tws_2/1
  BS_Req/3 -> Relational Operator1/1, Scope3/1  "<testSig_Rail_stBlkShtStM>"
  BS_Result/3 -> Relational Operator1/2, Scope3/2  "<Rail_stBlkShtStM>"
  Relational Operator1/1 -> AndN/3, Scope/3, tws_3/1

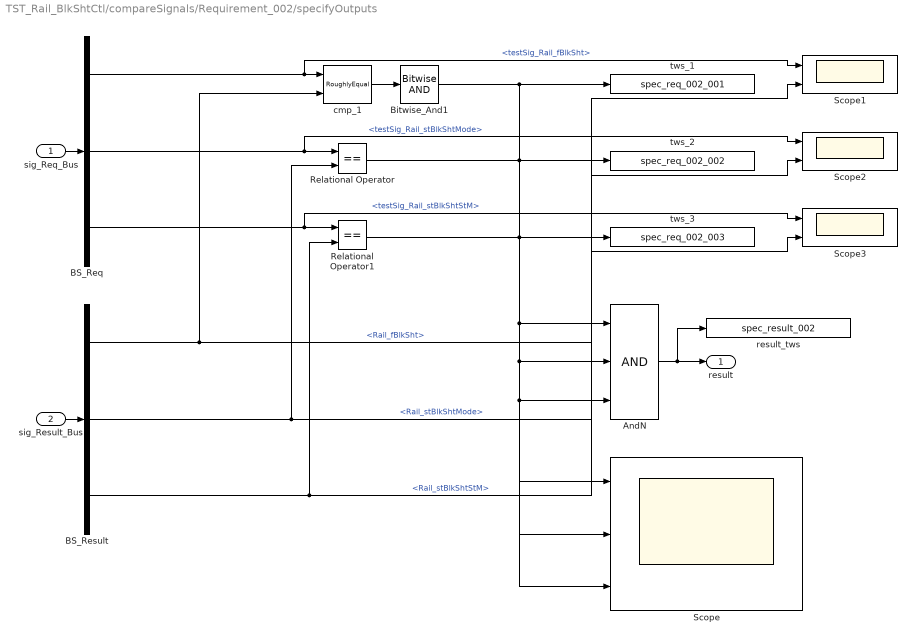
== system TST_Rail_BlkShtCtl/compareSignals/Requirement_002/specifyOutputs ==
  sig_Req_Bus : Inport
  sig_Result_Bus : Inport  Port=2
  AndN : Logic  Inputs=3
  BS_Req : BusSelector  OutputSignals=testSig_Rail_fBlkSht,testSig_Rail_stBlkShtMode,testSig_Rail_stBlkShtStM
  BS_Result : BusSelector  OutputSignals=Rail_fBlkSht,Rail_stBlkShtMode,Rail_stBlkShtStM
  Bitwise_And1 : simulink/Logic and Bit Operations/Bitwise Operator  logicop=AND  UseBitMask=off  BitMask=bin2dec('11011001')  BitMaskRealWorld=Stored Integer
  Relational Operator : RelationalOperator  Operator===  OutDataTypeStr=boolean  RndMeth=Simplest
  Relational Operator1 : RelationalOperator  Operator===  OutDataTypeStr=boolean  RndMeth=Simplest
  Scope : Scope  NumInputPorts=3
  Scope1 : Scope  NumInputPorts=2
  Scope2 : Scope  NumInputPorts=2
  Scope3 : Scope  NumInputPorts=2
  cmp_1 : UnitTest_Lib/RoughlyEqual  slope=0.1
  result_tws : ToWorkspace  VariableName=spec_result_002
  tws_1 : ToWorkspace  VariableName=spec_req_002_001
  tws_2 : ToWorkspace  VariableName=spec_req_002_002
  tws_3 : ToWorkspace  VariableName=spec_req_002_003
  result : Outport
  wires:
  sig_Req_Bus/1 -> BS_Req/1
  sig_Result_Bus/1 -> BS_Result/1
  AndN/1 -> result/1, result_tws/1
  BS_Req/1 -> cmp_1/1, Scope1/1  "<testSig_Rail_fBlkSht>"
  BS_Result/1 -> cmp_1/2, Scope1/2  "<Rail_fBlkSht>"
  cmp_1/1 -> Bitwise_And1/1
  Bitwise_And1/1 -> AndN/1, Scope/1, tws_1/1
  BS_Req/2 -> Relational Operator/1, Scope2/1  "<testSig_Rail_stBlkShtMode>"
  BS_Result/2 -> Scope2/2, Relational Operator/2  "<Rail_stBlkShtMode>"
  Relational Operator/1 -> AndN/2, Scope/2, tws_2/1
  BS_Req/3 -> Relational Operator1/1, Scope3/1  "<testSig_Rail_stBlkShtStM>"
  BS_Result/3 -> Relational Operator1/2, Scope3/2  "<Rail_stBlkShtStM>"
  Relational Operator1/1 -> AndN/3, Scope/3, tws_3/1

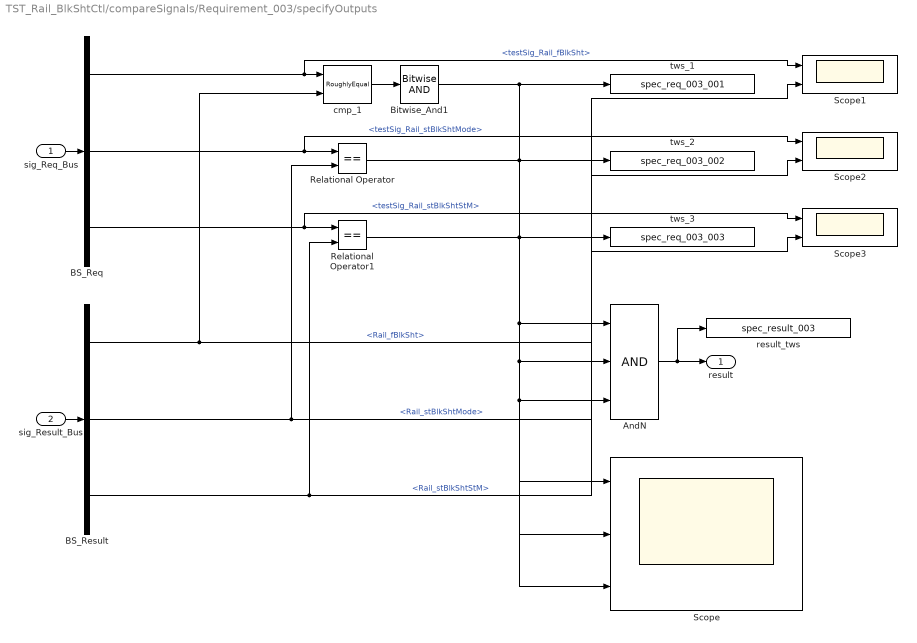
== system TST_Rail_BlkShtCtl/compareSignals/Requirement_003/specifyOutputs ==
  sig_Req_Bus : Inport
  sig_Result_Bus : Inport  Port=2
  AndN : Logic  Inputs=3
  BS_Req : BusSelector  OutputSignals=testSig_Rail_fBlkSht,testSig_Rail_stBlkShtMode,testSig_Rail_stBlkShtStM
  BS_Result : BusSelector  OutputSignals=Rail_fBlkSht,Rail_stBlkShtMode,Rail_stBlkShtStM
  Bitwise_And1 : simulink/Logic and Bit Operations/Bitwise Operator  logicop=AND  UseBitMask=off  BitMask=bin2dec('11011001')  BitMaskRealWorld=Stored Integer
  Relational Operator : RelationalOperator  Operator===  OutDataTypeStr=boolean  RndMeth=Simplest
  Relational Operator1 : RelationalOperator  Operator===  OutDataTypeStr=boolean  RndMeth=Simplest
  Scope : Scope  NumInputPorts=3
  Scope1 : Scope  NumInputPorts=2
  Scope2 : Scope  NumInputPorts=2
  Scope3 : Scope  NumInputPorts=2
  cmp_1 : UnitTest_Lib/RoughlyEqual  slope=0.1
  result_tws : ToWorkspace  VariableName=spec_result_003
  tws_1 : ToWorkspace  VariableName=spec_req_003_001
  tws_2 : ToWorkspace  VariableName=spec_req_003_002
  tws_3 : ToWorkspace  VariableName=spec_req_003_003
  result : Outport
  wires:
  sig_Req_Bus/1 -> BS_Req/1
  sig_Result_Bus/1 -> BS_Result/1
  AndN/1 -> result/1, result_tws/1
  BS_Req/1 -> cmp_1/1, Scope1/1  "<testSig_Rail_fBlkSht>"
  BS_Result/1 -> cmp_1/2, Scope1/2  "<Rail_fBlkSht>"
  cmp_1/1 -> Bitwise_And1/1
  Bitwise_And1/1 -> AndN/1, Scope/1, tws_1/1
  BS_Req/2 -> Relational Operator/1, Scope2/1  "<testSig_Rail_stBlkShtMode>"
  BS_Result/2 -> Scope2/2, Relational Operator/2  "<Rail_stBlkShtMode>"
  Relational Operator/1 -> AndN/2, Scope/2, tws_2/1
  BS_Req/3 -> Relational Operator1/1, Scope3/1  "<testSig_Rail_stBlkShtStM>"
  BS_Result/3 -> Relational Operator1/2, Scope3/2  "<Rail_stBlkShtStM>"
  Relational Operator1/1 -> AndN/3, Scope/3, tws_3/1
